simulink library "Propulsion"  (R2016a)
settings: Solver=ode45  StartTime=0.0  StopTime=10.0  RelTol=1e-3
values from neighbouring files (symbols this model uses):
  alfaf_deg = -1.8    [initACFT_high.m]
  nrho = 0.75    [initACFT_high.m]
  nv = 0    [initACFT_high.m]
  rho_reference_kgpm3 = 1.225    [initACFT_high.m]
  Tmax = 68000    [initACFT_high.m]
  V_reference_mps = 200    [initACFT_high.m]
  xf_m = -3.8    [initACFT_high.m]
  zf_m = -0.6    [initACFT_high.m]
settings Model: Creator=bruno  LastModifiedBy=bruno
settings DataIOCC: LimitDataPoints=on
settings DebuggingCC: AllowSymbolicDim=off

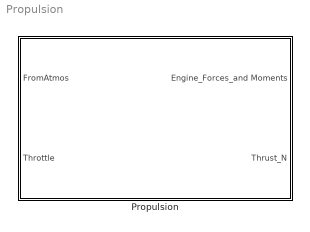
== system Propulsion ==
  Propulsion : Subsystem

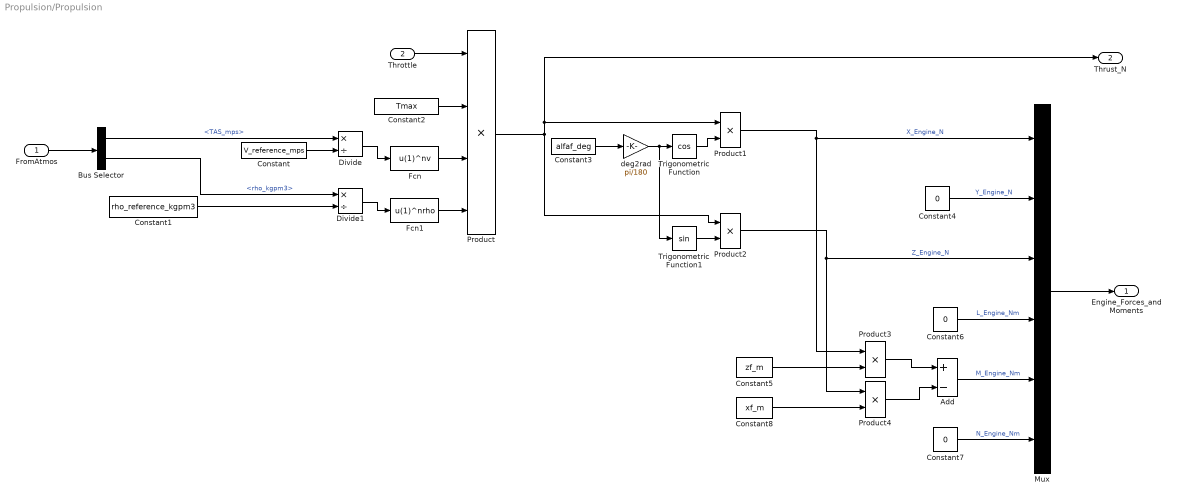
== system Propulsion/Propulsion ==
  FromAtmos : Inport
  Throttle : Inport  Port=2
  Add : Sum  Inputs=+-
  Bus Selector : BusSelector  OutputSignals=TAS_mps,rho_kgpm3
  Constant : Constant  Value=V_reference_mps
  Constant1 : Constant  Value=rho_reference_kgpm3
  Constant2 : Constant  Value=Tmax
  Constant3 : Constant  Value=alfaf_deg
  Constant4 : Constant  Value=0
  Constant5 : Constant  Value=zf_m
  Constant6 : Constant  Value=0
  Constant7 : Constant  Value=0
  Constant8 : Constant  Value=xf_m
  Divide : Product  Inputs=*/
  Divide1 : Product  Inputs=*/
  Fcn : Fcn  Expr=u(1)^nv
  Fcn1 : Fcn  Expr=u(1)^nrho
  Mux : Mux  Inputs=6
  Product : Product  Inputs=4
  Product{1..4} (4 alike) : Product
  Trigonometric Function : Trigonometry  Operator=cos
  Trigonometric Function1 : Trigonometry
  deg2rad : Gain  Gain=pi/180
  Engine_Forces_and Moments : Outport
  Thrust_N : Outport  Port=2
  wires:
  Trigonometric Function1/1 -> Product2/2
  Throttle/1 -> Product/1
  Constant/1 -> Divide/2
  Product3/1 -> Add/1
  Constant1/1 -> Divide1/2
  Divide1/1 -> Fcn1/1
  Constant5/1 -> Product3/2
  Constant3/1 -> deg2rad/1
  Product4/1 -> Add/2
  Constant6/1 -> Mux/4  "L_Engine_Nm"
  Fcn1/1 -> Product/4
  Constant7/1 -> Mux/6  "N_Engine_Nm"
  Bus Selector/2 -> Divide1/1  "<rho_kgpm3>"
  Fcn/1 -> Product/3
  Constant2/1 -> Product/2
  Divide/1 -> Fcn/1
  FromAtmos/1 -> Bus Selector/1
  Product2/1 -> Mux/3, Product4/1  "Z_Engine_N"
  Mux/1 -> Engine_Forces_and Moments/1
  Product/1 -> Product2/1, Thrust_N/1, Product1/1
  deg2rad/1 -> Trigonometric Function1/1, Trigonometric Function/1
  Product1/1 -> Mux/1, Product3/1  "X_Engine_N"
  Trigonometric Function/1 -> Product1/2
  Constant4/1 -> Mux/2  "Y_Engine_N"
  Constant8/1 -> Product4/2
  Add/1 -> Mux/5  "M_Engine_Nm"
  Bus Selector/1 -> Divide/1  "<TAS_mps>"
